simulink model "changer"  (Simulink 5.0)
settings: Solver=ode45  StartTime=0.0  StopTime=10.0  RelTol=1e-3
settings Model: LastModifiedBy=dsplab

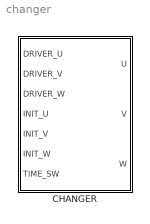
== system changer ==
  CHANGER : Subsystem  mask{T=0}
      mask prompts: T "Threshold time"

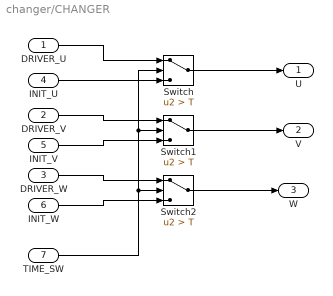
== system changer/CHANGER ==
  DRIVER_U : Inport
  DRIVER_V : Inport  Port=2
  DRIVER_W : Inport  Port=3
  INIT_U : Inport  Port=4
  INIT_V : Inport  Port=5
  INIT_W : Inport  Port=6
  TIME_SW : Inport  Port=7
  Switch : Switch  Criteria=u2 > Threshold  Threshold=T  SaturateOnIntegerOverflow=on
  Switch1 : Switch  Criteria=u2 > Threshold  Threshold=T  SaturateOnIntegerOverflow=on
  Switch2 : Switch  Criteria=u2 > Threshold  Threshold=T  SaturateOnIntegerOverflow=on
  U : Outport
  V : Outport  Port=2
  W : Outport  Port=3
  wires:
  DRIVER_U/1 -> Switch/1
  DRIVER_V/1 -> Switch1/1
  DRIVER_W/1 -> Switch2/1
  INIT_U/1 -> Switch/3
  INIT_V/1 -> Switch1/3
  INIT_W/1 -> Switch2/3
  TIME_SW/1 -> Switch/2, Switch1/2, Switch2/2
  Switch2/1 -> W/1
  Switch1/1 -> V/1
  Switch/1 -> U/1
